simulink model "actuators_subsytem"  (R2024a)
settings: Solver=VariableStepAuto  StartTime=0.0  StopTime=10.0  RelTol=1e-3
settings Model: Creator=adity  LastModifiedBy=adity

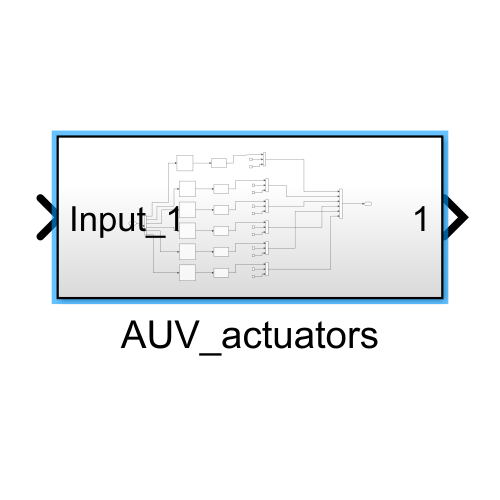
[thumbnail: Simulink's stored preview of the top-level diagram]
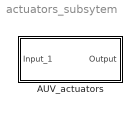
== system actuators_subsytem ==
  AUV_actuators : Subsystem

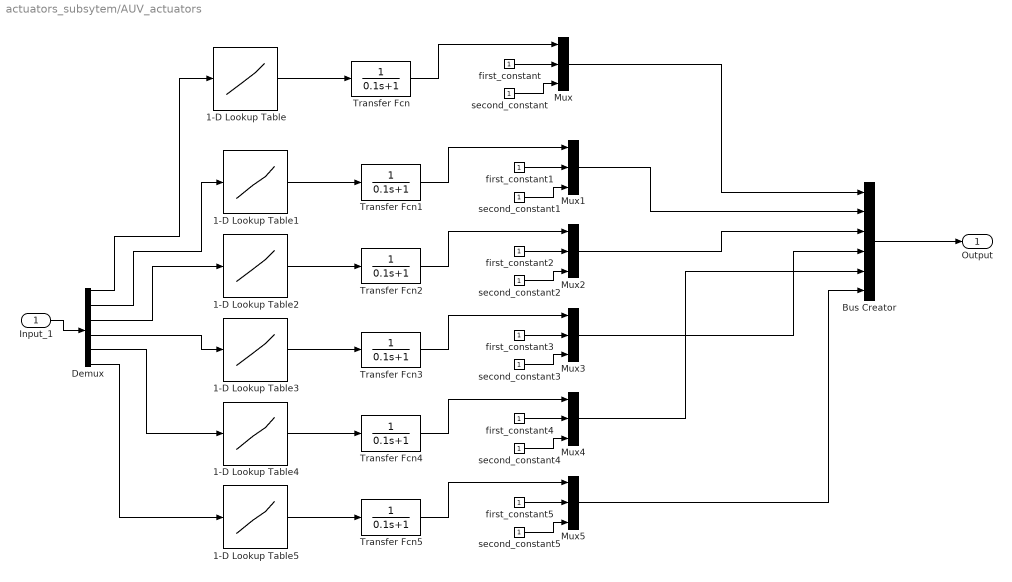
== system actuators_subsytem/AUV_actuators ==
  Input_1 : Inport
  1-D Lookup Table{,1..5} (6 alike) : Lookup_n-D  NumberOfTableDimensions=1  BreakpointsForDimension1=[-1,-0.1,0,0.1,1]  Table=[-40,-1,0,1,50]  InternalRulePriority=Speed  RndMeth=Simplest
  Bus Creator : BusCreator  Inputs=6
  Demux : Demux  Outputs=6
  Mux{,1..5} (6 alike) : Mux  Inputs=3
  Transfer Fcn{,1..5} (6 alike) : TransferFcn  Denominator=[0.1 1]
  first_constant{,1..5} (6 alike) : Constant
  second_constant{,1..5} (6 alike) : Constant
  Output : Outport
  wires:
  Demux/1 -> 1-D Lookup Table/1
  1-D Lookup Table/1 -> Transfer Fcn/1
  Transfer Fcn/1 -> Mux/1
  first_constant/1 -> Mux/2
  second_constant/1 -> Mux/3
  first_constant1/1 -> Mux1/2
  1-D Lookup Table1/1 -> Transfer Fcn1/1
  second_constant1/1 -> Mux1/3
  Demux/2 -> 1-D Lookup Table1/1
  Transfer Fcn1/1 -> Mux1/1
  Transfer Fcn2/1 -> Mux2/1
  second_constant2/1 -> Mux2/3
  first_constant2/1 -> Mux2/2
  1-D Lookup Table2/1 -> Transfer Fcn2/1
  Demux/3 -> 1-D Lookup Table2/1
  Transfer Fcn3/1 -> Mux3/1
  second_constant3/1 -> Mux3/3
  first_constant3/1 -> Mux3/2
  1-D Lookup Table3/1 -> Transfer Fcn3/1
  Demux/4 -> 1-D Lookup Table3/1
  Transfer Fcn4/1 -> Mux4/1
  second_constant4/1 -> Mux4/3
  first_constant4/1 -> Mux4/2
  1-D Lookup Table4/1 -> Transfer Fcn4/1
  Demux/5 -> 1-D Lookup Table4/1
  Transfer Fcn5/1 -> Mux5/1
  second_constant5/1 -> Mux5/3
  first_constant5/1 -> Mux5/2
  1-D Lookup Table5/1 -> Transfer Fcn5/1
  Demux/6 -> 1-D Lookup Table5/1
  Mux/1 -> Bus Creator/1
  Mux1/1 -> Bus Creator/2
  Mux2/1 -> Bus Creator/3
  Mux3/1 -> Bus Creator/4
  Mux4/1 -> Bus Creator/5
  Mux5/1 -> Bus Creator/6
  Input_1/1 -> Demux/1
  Bus Creator/1 -> Output/1
